simulink library "Lib_Solve_PWLinearize_TMATS"  (R2019b)
settings: Solver=ode45  StartTime=0.0  StopTime=10.0  RelTol=1e-3  EnableMultiTasking=on
libraries: simulink x8, Lib_Solve_Linearize_TMATS x1, Lib_Cntrl_SetPointCntrlPI_TMATS x1, Lib_Solve_OuterLoopIntegrator_TMATS x1
Description:
  | Thomas Modules
settings Model: Creator=jwchapm2  LastModifiedBy=bhisma
settings DataIOCC: LimitDataPoints=on  SaveFormat=Array  ReturnWorkspaceOutputs=off
settings OptimizationCC: ExpressionDepthLimit=2147483647  LifeSpan=inf
settings DebuggingCC: UnderspecifiedInitializationDetection=Classic  MergeDetectMultiDrivingBlocksExec=none  SolverPrmCheckMsg=warning  StateNameClashWarn=warning  SFUnexpectedBacktrackingDiag=warning  SFNoUnconditionalDefaultTransitionDiag=warning  SFExecutionAtInitializationDiag=none  ArithmeticOperatorsInVariantConditions=warning
settings HardwareCC: ProdBitPerPointer=32  ProdBitPerSizeT=32  ProdBitPerPtrDiffT=32  ProdLargestAtomicFloat=None  ProdIntDivRoundTo=Undefined  ProdEndianess=Unspecified  ProdWordSize=32  ProdHWDeviceType=32-bit Generic
settings ModelReferenceCC: PropagateSignalLabelsOutOfModel=off
settings SFSimCC: SimUseLocalCustomCode=off  CustomCodeUndefinedFunction=UseInterfaceOnly
settings RTWCC: RTWUseLocalCustomCode=off
settings CodeAppCC: StateflowObjectComments=on
settings GRTTargetCC: TargetLangStandard=C89/C90 (ANSI)  GeneratePreprocessorConditionals=Disable all
settings ConfigComp: CovMetricSettings=dw  CovHtmlReporting=on  CovSaveCumulativeToWorkspaceVar=on  CovSaveSingleToWorkspaceVar=on  CovExternalEMLEnable=off

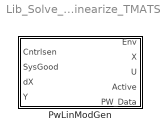
== system Lib_Solve_PWLinearize_TMATS ==
  PwLinModGen : Subsystem  mask(T-MATS: Piecewise Linear Model Generator Library Block){Env_M=[0 100 1000;0 0.05 0.1], DCntrlEn_M=off, TVec_M=0: 50: 100, XIC_M=[7000; 10000], UIC_M=10000, Ts_M=0.015, Kp_M=0.001, Ki_M=0.001, ER_M=[100; 0.001], UR_M=2, dXC_M=0.001, Fail_M=2, XPer_M=[0.01;-0.01], UPer_M=[0.01;-0.01], NY_M=8, BN_M=double(gcb)}
      mask prompts: Env_M "Env_M - Environmental Parameter Array (mxn)"; DCntrlEn_M "DCntrlEn_M - Enable direct U control"; TVec_M "TVec_M - Target control value or direct U vector (rx1)"; XIC_M "XIC_M - Initial conditions for system states (px1)"; UIC_M "UIC_M - Initial conditions for U (1x1)"; Ts_M "Ts_M - Sample time"; ER_M "ER_M - quasi-steady-state environmental parameter slew rate (mx1)"; UR_M "UR_M - quasi-steady-state U slew rate (1x1)"; dXC_M "dXC_M - dX steady-state conditional limit"; Fail_M "Fail_M - Time required to fail slew run (sec)"; XPer_M "XPer_M - X perturbation values (rxm) [frac]"; UPer_M "UPer_M - U perturbation values (rx1) [frac]"; NY_M "NY_M - Number of Y variables"; BN_M "BN_M - Block Name"
      mask help:
      | This block is meant to automatically create a piecewise linear model of a system.
      |
      | This model will be of the form:
      | (xdot - xdot_0) = A*(x - x0) + B*(u - u0)
      | (y - y0) = C*(x - x0) + D*(u - u0)
      |
      | Where x is the system state, u is the system input, and y is the plant output.
      | 0 values are the trim point values.
      |
      | This block should only be used when U is a 1x1 and the system states are external.
      |
      | During operation, the block will dynamically move or "slew" the system input and various environmental inputs to the defined operational points. At these points the block will wait for the system to reach steady state, then freeze the state integrators while the system is linearized using the perturbation method (see the T-MATS linearization block). As points are linearized, the block will output the linear models to the file "LinPW_TMATS.mat". Control of u slew rates can be managed in two ways. First with a direct dynamic slew of u (check box DCntrlEn_M) and second with by using u as an effector to meet a desired control value. The control value can be input into the Cntrlsen input and u is adjusted via a proportional integral (PI) controller to move the system to the desired control value.
      | For more information click on the help button.
      mask init:
      | if DCntrlEn_M == 0
      |     if strcmp(get_param([BN_M '/Cntrlsen'],'BlockType'),'Constant')
      |         MSK_ReplaceBlock_TMATS([BN_M '/Cntrlsen'],'built-in/Inport');
      |     end
      |     set_param([BN_M '/Cntrlsen'],'Port',num2str(1));
      | elseif DCntrlEn_M == 1
      |     if strcmp(get_param([BN_M '/Cntrlsen'],'BlockType'),'Inport')
      |         MSK_ReplaceBlock_TMATS([BN_M '/Cntrlsen'],'built-in/Constant');
      |         set_param([BN_M '/Cntrlsen'],'Value','[0]');
      |     end
      | end
      mask Help: web(which('Solver_TMATS_PWLinearize.html'),'-helpbrowser')
      mask Callback DCntrlEn_M: MSK_SEC_Enables_TMATS('DCntrlEn_M',[7,8],'dis')
      mask DialogControl Container4 Prompt: Slew
      mask DialogControl Container7 Prompt: SlewCntrl
      mask DialogControl Container5 Prompt: Linearization

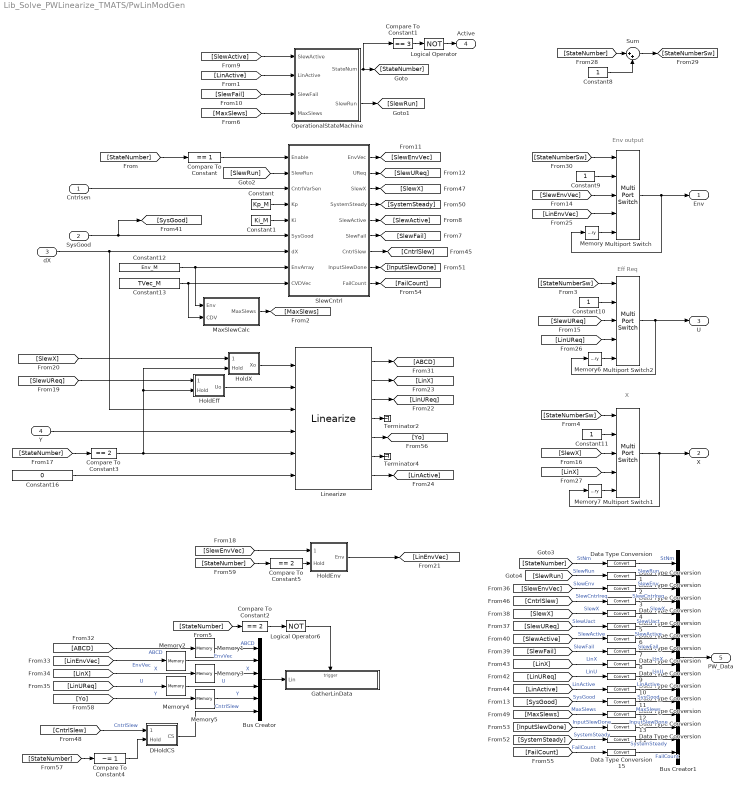
== system Lib_Solve_PWLinearize_TMATS/PwLinModGen ==
  note: X
  note: Eff Req
  note: Env output
  Cntrlsen : Inport
  SysGood : Inport  Port=2
  dX : Inport  Port=3
  Y : Inport  Port=4
  Bus Creator : BusCreator  Inputs=6
  Bus Creator1 : BusCreator  Inputs=16
  Compare To Constant : simulink/Logic and Bit Operations/Compare To Constant  relop===  const=1  OutDataTypeStr=boolean
  Compare To Constant1 : simulink/Logic and Bit Operations/Compare To Constant  relop===  const=3  OutDataTypeStr=boolean
  Compare To Constant2 : simulink/Logic and Bit Operations/Compare To Constant  relop===  const=2  OutDataTypeStr=boolean
  Compare To Constant3 : simulink/Logic and Bit Operations/Compare To Constant  relop===  const=2  OutDataTypeStr=boolean
  Compare To Constant4 : simulink/Logic and Bit Operations/Compare To Constant  relop=~=  const=1  OutDataTypeStr=boolean
  Compare To Constant5 : simulink/Logic and Bit Operations/Compare To Constant  relop===  const=2  OutDataTypeStr=boolean
  Constant : Constant  Value=Kp_M
  Constant1 : Constant  Value=Ki_M
  Constant{8..11} (4 alike) : Constant
  Constant12 : Constant  Value=Env_M
  Constant13 : Constant  Value=TVec_M
  Constant16 : Constant  Value=0
  DHoldCS : Subsystem
  Data Type Conversion{,1..15} (16 alike) : DataTypeConversion
  GatherLinData : Subsystem
  HoldEff : Subsystem
  HoldEnv : Subsystem
  HoldX : Subsystem
  Linearize : Lib_Solve_Linearize_TMATS/Linearize  N_XPer_M=XPer_M  N_UPer_M=UPer_M  N_Y_M=NY_M
  Logical Operator : Logic  Operator=NOT  AllPortsSameDT=off  OutDataTypeStr=boolean
  Logical Operator6 : Logic  Operator=NOT  AllPortsSameDT=off  OutDataTypeStr=boolean
  MaxSlewCalc : Subsystem
  Memory : Memory  InitialCondition=Env_M(:,1)
  Memory{1..5} (5 alike) : Memory
  Memory6 : Memory  InitialCondition=UIC_M
  Memory7 : Memory  InitialCondition=XIC_M
  Multiport Switch : MultiPortSwitch  Inputs=4
  Multiport Switch1 : MultiPortSwitch  Inputs=4
  Multiport Switch2 : MultiPortSwitch  Inputs=4
  OperationalStateMachine : Subsystem  TreatAsAtomicUnit=on
  SlewCntrl : Subsystem
  Sum : Sum  Inputs=|++
  Terminator2 : Terminator
  Terminator4 : Terminator
  Env : Outport  PortDimensions=size(Env_M,1)
  X : Outport  Port=2  PortDimensions=length(XIC_M)
  U : Outport  Port=3  PortDimensions=length(UIC_M)
  Active : Outport  Port=4
  PW_Data : Outport  Port=5
  wires:
  Bus Creator/1 -> GatherLinData/1(Lin)
  [LinUReq] -> Memory4/1  "U"
  [ABCD] -> Memory1/1  "ABCD"
  [LinEnvVec] -> Memory2/1  "EnvVec"
  [LinX] -> Memory3/1  "X"
  Logical Operator6/1 -> GatherLinData/Trigger
  [StateNumber] -> Compare To Constant2/1
  Compare To Constant2/1 -> Logical Operator6/1
  Logical Operator/1 -> Active/1
  Compare To Constant1/1 -> Logical Operator/1
  SlewCntrl/1(EnvVec) -> [SlewEnvVec]
  [SlewX] -> HoldX/1(SlewX)
  [StateNumber] -> Sum/1
  Memory7/1 -> Multiport Switch1/5
  Constant11/1 -> Multiport Switch1/2
  Constant10/1 -> Multiport Switch2/2
  [SlewUReq] -> Multiport Switch2/3
  Memory6/1 -> Multiport Switch2/5
  Memory/1 -> Multiport Switch/5
  [LinUReq] -> Multiport Switch2/4
  Constant9/1 -> Multiport Switch/2
  [SlewUReq] -> HoldEff/1(SlewU)
  Multiport Switch1/1 -> Memory7/1, X/1
  [StateNumber] -> Compare To Constant/1
  [StateNumberSw] -> Multiport Switch1/1
  [StateNumberSw] -> Multiport Switch2/1
  [StateNumberSw] -> Multiport Switch/1
  OperationalStateMachine/1(StateNum) -> [StateNumber], Compare To Constant1/1
  Constant13/1 -> MaxSlewCalc/2(CDV), SlewCntrl/9(CVDVec)
  Constant12/1 -> MaxSlewCalc/1(Env), SlewCntrl/8(EnvArray)
  MaxSlewCalc/1(MaxSlews) -> [MaxSlews]
  dX/1 -> Linearize/3, SlewCntrl/7(dX)
  Constant16/1 -> Linearize/6
  Y/1 -> Linearize/4
  Constant8/1 -> Sum/2
  Sum/1 -> [StateNumberSw]
  [MaxSlews] -> OperationalStateMachine/4(MaxSlews)
  Linearize/1 -> [ABCD]
  Linearize/6 -> Terminator4/1
  Linearize/5 -> [Yo]
  Linearize/4 -> Terminator2/1
  Compare To Constant3/1 -> Linearize/5, HoldX/2(Hold), HoldEff/2(Hold)
  SysGood/1 -> [SysGood], SlewCntrl/6(SysGood)
  SlewCntrl/2(UReq) -> [SlewUReq]
  [SlewActive] -> OperationalStateMachine/1(SlewActive)
  [StateNumber] -> Compare To Constant3/1
  Linearize/7 -> [LinActive]
  [LinActive] -> OperationalStateMachine/2(LinActive)
  [SlewEnvVec] -> Multiport Switch/3
  OperationalStateMachine/2(SlewRun) -> [SlewRun]
  [LinX] -> Multiport Switch1/4
  SlewCntrl/5(SlewActive) -> [SlewActive]
  Multiport Switch2/1 -> Memory6/1, U/1
  [SlewFail] -> OperationalStateMachine/3(SlewFail)
  SlewCntrl/6(SlewFail) -> [SlewFail]
  HoldEff/1(Uo) -> Linearize/2
  [SlewRun] -> SlewCntrl/2(SlewRun)
  Cntrlsen/1 -> SlewCntrl/3(CntrlVarSen)
  [SlewX] -> Multiport Switch1/3
  Constant1/1 -> SlewCntrl/5(Ki)
  SlewCntrl/4(SystemSteady) -> [SystemSteady]
  Constant/1 -> SlewCntrl/4(Kp)
  Linearize/2 -> [LinX]
  [LinEnvVec] -> Multiport Switch/4
  HoldEnv/1(Env) -> [LinEnvVec]
  Linearize/3 -> [LinUReq]
  Multiport Switch/1 -> Memory/1, Env/1
  [CntrlSlew] -> Data Type Conversion3/1  "SlewCntrlreq"
  [SlewRun] -> Data Type Conversion1/1  "SlewRun"
  [SlewEnvVec] -> Data Type Conversion2/1  "SlewEnv"
  [SlewX] -> Data Type Conversion4/1  "SlewX"
  [StateNumber] -> Data Type Conversion/1  "StNm"
  [LinX] -> Data Type Conversion8/1  "LinX"
  [SlewUReq] -> Data Type Conversion5/1  "SlewUact"
  [LinActive] -> Data Type Conversion10/1  "LinActive"
  [SlewFail] -> Data Type Conversion7/1  "SlewFail"
  [LinUReq] -> Data Type Conversion9/1  "LinU"
  [SlewActive] -> Data Type Conversion6/1  "SlewActive"
  Bus Creator1/1 -> PW_Data/1
  Compare To Constant/1 -> SlewCntrl/1(Enable)
  SlewCntrl/3(SlewX) -> [SlewX]
  [SysGood] -> Data Type Conversion11/1  "SysGood"
  [CntrlSlew] -> DHoldCS/1(CntrlSlew)  "CntrlSlew"
  [MaxSlews] -> Data Type Conversion12/1  "MaxSlews"
  SlewCntrl/8(InputSlewDone) -> [InputSlewDone]
  [InputSlewDone] -> Data Type Conversion13/1  "InputSlewDone"
  [SystemSteady] -> Data Type Conversion14/1  "SystemSteady"
  SlewCntrl/9(FailCount) -> [FailCount]
  [FailCount] -> Data Type Conversion15/1  "FailCount"
  HoldX/1(Xo) -> Linearize/1
  [Yo] -> Memory5/1  "Y"
  Memory1/1 -> Bus Creator/1  "ABCD"
  Memory2/1 -> Bus Creator/2  "EnvVec"
  Memory3/1 -> Bus Creator/3  "X"
  Memory4/1 -> Bus Creator/4  "U"
  Memory5/1 -> Bus Creator/5  "Y"
  DHoldCS/1(CS) -> Bus Creator/6  "CntrlSlew"
  SlewCntrl/7(CntrlSlew) -> [CntrlSlew]
  [StateNumber] -> Compare To Constant4/1
  Compare To Constant4/1 -> DHoldCS/2(Hold)
  Data Type Conversion/1 -> Bus Creator1/1  "StNm"
  Data Type Conversion1/1 -> Bus Creator1/2  "SlewRun"
  Data Type Conversion2/1 -> Bus Creator1/3  "SlewEnv"
  Data Type Conversion3/1 -> Bus Creator1/4  "SlewCntrlreq"
  Data Type Conversion4/1 -> Bus Creator1/5  "SlewX"
  Data Type Conversion5/1 -> Bus Creator1/6  "SlewUact"
  Data Type Conversion6/1 -> Bus Creator1/7  "SlewActive"
  Data Type Conversion7/1 -> Bus Creator1/8  "SlewFail"
  Data Type Conversion8/1 -> Bus Creator1/9  "LinX"
  Data Type Conversion9/1 -> Bus Creator1/10  "LinU"
  Data Type Conversion10/1 -> Bus Creator1/11  "LinActive"
  Data Type Conversion11/1 -> Bus Creator1/12  "SysGood"
  Data Type Conversion12/1 -> Bus Creator1/13  "MaxSlews"
  Data Type Conversion13/1 -> Bus Creator1/14  "InputSlewDone"
  Data Type Conversion14/1 -> Bus Creator1/15  "SystemSteady"
  Data Type Conversion15/1 -> Bus Creator1/16  "FailCount"
  [SlewEnvVec] -> HoldEnv/1(SlewEnv)
  [StateNumber] -> Compare To Constant5/1
  Compare To Constant5/1 -> HoldEnv/2(Hold)

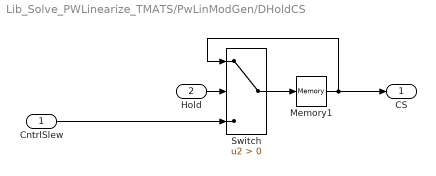
== system Lib_Solve_PWLinearize_TMATS/PwLinModGen/DHoldCS ==
  CntrlSlew : Inport
  Hold : Inport  Port=2
  Memory1 : Memory  InitialCondition=TVec_M(1)
  Switch : Switch  Criteria=u2 > Threshold
  CS : Outport
  wires:
  CntrlSlew/1 -> Switch/3
  Memory1/1 -> Switch/1, CS/1
  Hold/1 -> Switch/2
  Switch/1 -> Memory1/1

== system Lib_Solve_PWLinearize_TMATS/PwLinModGen/GatherLinData ==
  Lin : Inport
  Trigger : TriggerPort  VariantControl=(inherit)  PortDimensions=1
  To File : ToFile  Filename=LinPW_TMATS  MatrixName=LinSys  SaveFormat=Timeseries
  wires:
  Lin/1 -> To File/1

== system Lib_Solve_PWLinearize_TMATS/PwLinModGen/HoldEff ==
  SlewU : Inport
  Hold : Inport  Port=2
  Memory2 : Memory  InitialCondition=UIC_M
  Switch : Switch  Criteria=u2 > Threshold
  Uo : Outport
  wires:
  Switch/1 -> Memory2/1, Uo/1
  Hold/1 -> Switch/2
  Memory2/1 -> Switch/1
  SlewU/1 -> Switch/3

== system Lib_Solve_PWLinearize_TMATS/PwLinModGen/HoldEnv ==
  SlewEnv : Inport
  Hold : Inport  Port=2
  Memory2 : Memory  InitialCondition=Env_M(:,1)
  Switch : Switch  Criteria=u2 > Threshold
  Env : Outport
  wires:
  SlewEnv/1 -> Switch/3
  Memory2/1 -> Switch/1
  Hold/1 -> Switch/2
  Switch/1 -> Env/1, Memory2/1

== system Lib_Solve_PWLinearize_TMATS/PwLinModGen/HoldX ==
  SlewX : Inport
  Hold : Inport  Port=2
  Memory2 : Memory  InitialCondition=XIC_M
  Switch : Switch  Criteria=u2 > Threshold
  Xo : Outport
  wires:
  Memory2/1 -> Switch/1
  Hold/1 -> Switch/2
  SlewX/1 -> Switch/3
  Switch/1 -> Memory2/1, Xo/1

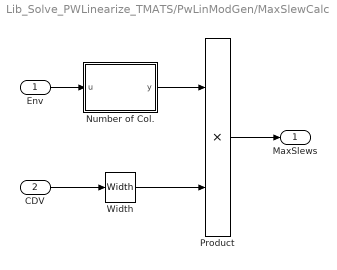
== system Lib_Solve_PWLinearize_TMATS/PwLinModGen/MaxSlewCalc ==
  Env : Inport
  CDV : Inport  Port=2
  Number of Col. : MATLAB Function  TreatAsAtomicUnit=on
  Product : Product
  Width : Width
  MaxSlews : Outport
  wires:
  CDV/1 -> Width/1
  Env/1 -> Number of Col./1(u)
  Number of Col./1(y) -> Product/1
  Product/1 -> MaxSlews/1
  Width/1 -> Product/2

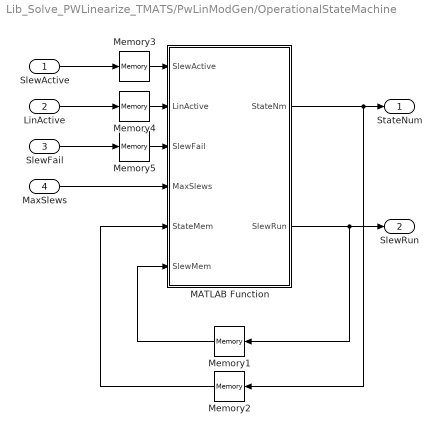
== system Lib_Solve_PWLinearize_TMATS/PwLinModGen/OperationalStateMachine ==
  SlewActive : Inport
  LinActive : Inport  Port=2
  SlewFail : Inport  Port=3
  MaxSlews : Inport  Port=4
  MATLAB Function : MATLAB Function  TreatAsAtomicUnit=on
  Memory1 : Memory  InitialCondition=1
  Memory{2..5} (4 alike) : Memory
  StateNum : Outport
  SlewRun : Outport  Port=2
  wires:
  MaxSlews/1 -> MATLAB Function/4(MaxSlews)
  Memory4/1 -> MATLAB Function/2(LinActive)
  LinActive/1 -> Memory4/1
  Memory5/1 -> MATLAB Function/3(SlewFail)
  Memory3/1 -> MATLAB Function/1(SlewActive)
  SlewFail/1 -> Memory5/1
  SlewActive/1 -> Memory3/1
  Memory1/1 -> MATLAB Function/6(SlewMem)
  MATLAB Function/2(SlewRun) -> SlewRun/1, Memory1/1
  MATLAB Function/1(StateNm) -> Memory2/1, StateNum/1
  Memory2/1 -> MATLAB Function/5(StateMem)

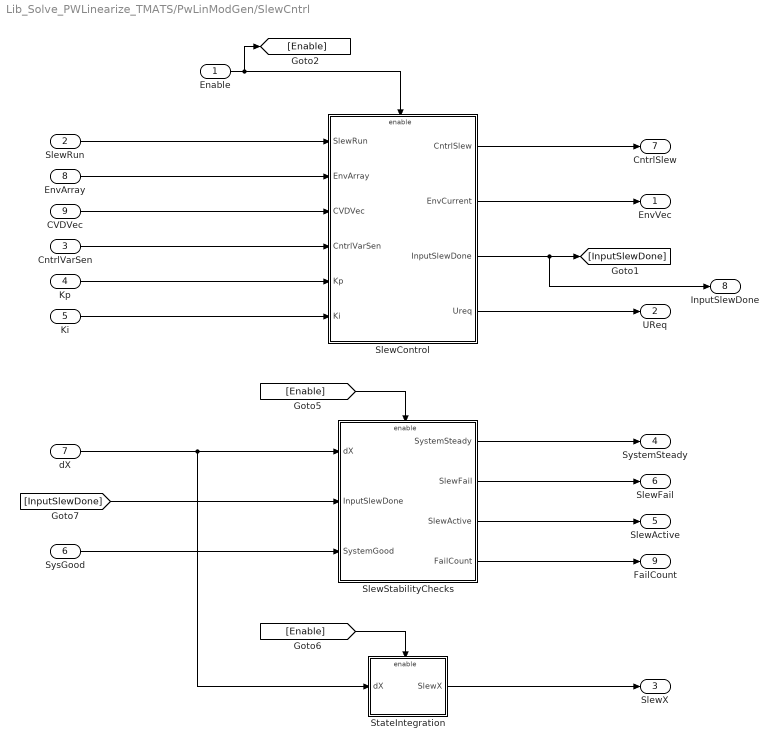
== system Lib_Solve_PWLinearize_TMATS/PwLinModGen/SlewCntrl ==
  Enable : Inport
  SlewRun : Inport  Port=2
  CntrlVarSen : Inport  Port=3
  Kp : Inport  Port=4
  Ki : Inport  Port=5
  SysGood : Inport  Port=6
  dX : Inport  Port=7
  EnvArray : Inport  Port=8
  CVDVec : Inport  Port=9
  SlewControl : Subsystem
  SlewStabilityChecks : Subsystem
  StateIntegration : Subsystem
  EnvVec : Outport
  UReq : Outport  Port=2
  SlewX : Outport  Port=3
  SystemSteady : Outport  Port=4
  SlewActive : Outport  Port=5
  SlewFail : Outport  Port=6
  CntrlSlew : Outport  Port=7
  InputSlewDone : Outport  Port=8
  FailCount : Outport  Port=9
  wires:
  SlewRun/1 -> SlewControl/1(SlewRun)
  EnvArray/1 -> SlewControl/2(EnvArray)
  CVDVec/1 -> SlewControl/3(CVDVec)
  CntrlVarSen/1 -> SlewControl/4(CntrlVarSen)
  Kp/1 -> SlewControl/5(Kp)
  Ki/1 -> SlewControl/6(Ki)
  SlewControl/1(CntrlSlew) -> CntrlSlew/1
  SlewControl/2(EnvCurrent) -> EnvVec/1
  SlewControl/3(InputSlewDone) -> InputSlewDone/1, [InputSlewDone]
  SlewControl/4(Ureq) -> UReq/1
  dX/1 -> StateIntegration/1(dX), SlewStabilityChecks/1(dX)
  [InputSlewDone] -> SlewStabilityChecks/2(InputSlewDone)
  SysGood/1 -> SlewStabilityChecks/3(SystemGood)
  SlewStabilityChecks/1(SystemSteady) -> SystemSteady/1
  SlewStabilityChecks/2(SlewFail) -> SlewFail/1
  SlewStabilityChecks/3(SlewActive) -> SlewActive/1
  Enable/1 -> SlewControl/Enable, [Enable]
  [Enable] -> SlewStabilityChecks/Enable
  [Enable] -> StateIntegration/Enable
  StateIntegration/1(SlewX) -> SlewX/1
  SlewStabilityChecks/4(FailCount) -> FailCount/1

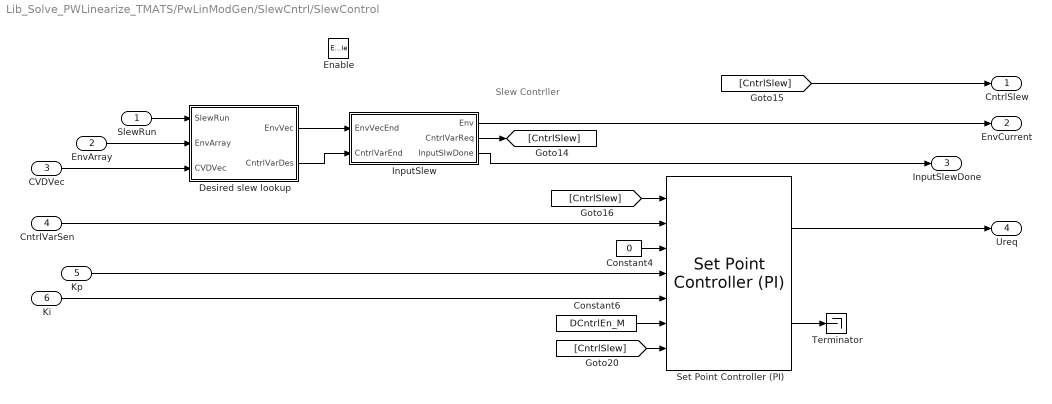
== system Lib_Solve_PWLinearize_TMATS/PwLinModGen/SlewCntrl/SlewControl ==
  note: Slew Contrller
  SlewRun : Inport
  EnvArray : Inport  Port=2
  CVDVec : Inport  Port=3
  CntrlVarSen : Inport  Port=4
  Kp : Inport  Port=5
  Ki : Inport  Port=6
  Enable : EnablePort
  Constant4 : Constant  Value=0
  Constant6 : Constant  Value=DCntrlEn_M
  Desired slew lookup : Subsystem
  InputSlew : Subsystem
  Set Point Controller (PI) : Lib_Cntrl_SetPointCntrlPI_TMATS/Set Point Controller (PI)  PI_IC_M=UIC_M  WGain_M=0  Ts_M=Ts_M
  Terminator : Terminator
  CntrlSlew : Outport
  EnvCurrent : Outport  Port=2
  InputSlewDone : Outport  Port=3
  Ureq : Outport  Port=4
  wires:
  Constant4/1 -> Set Point Controller (PI)/3
  CVDVec/1 -> Desired slew lookup/3(CVDVec)
  SlewRun/1 -> Desired slew lookup/1(SlewRun)
  Desired slew lookup/1(EnvVec) -> InputSlew/1(EnvVecEnd)
  Kp/1 -> Set Point Controller (PI)/4
  InputSlew/3(InputSlwDone) -> InputSlewDone/1
  Desired slew lookup/2(CntrlVarDes) -> InputSlew/2(CntrlVarEnd)
  CntrlVarSen/1 -> Set Point Controller (PI)/2
  Ki/1 -> Set Point Controller (PI)/5
  InputSlew/1(Env) -> EnvCurrent/1
  Set Point Controller (PI)/1 -> Ureq/1
  Constant6/1 -> Set Point Controller (PI)/6
  [CntrlSlew] -> Set Point Controller (PI)/7
  Set Point Controller (PI)/2 -> Terminator/1
  InputSlew/2(CntrlVarReq) -> [CntrlSlew]
  [CntrlSlew] -> CntrlSlew/1
  [CntrlSlew] -> Set Point Controller (PI)/1
  EnvArray/1 -> Desired slew lookup/2(EnvArray)

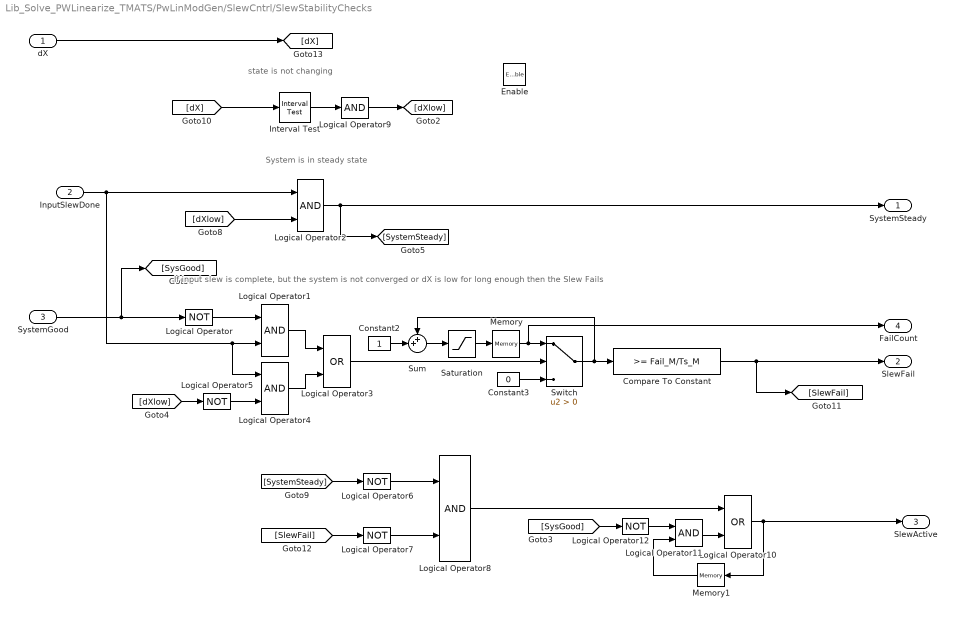
== system Lib_Solve_PWLinearize_TMATS/PwLinModGen/SlewCntrl/SlewStabilityChecks ==
  note: state is not changing
  note: If input slew is complete, but the system is not converged or dX is low for long enough then the Slew Fails
  note: System is in steady state
  dX : Inport
  InputSlewDone : Inport  Port=2
  SystemGood : Inport  Port=3
  Enable : EnablePort
  Compare To Constant : simulink/Logic and Bit Operations/Compare To Constant  relop=>=  const=Fail_M/Ts_M  OutDataTypeStr=boolean
  Constant2 : Constant
  Constant3 : Constant  Value=0
  Interval Test : simulink/Logic and Bit Operations/Interval Test  IntervalClosedRight=on  uplimit=dXC_M  IntervalClosedLeft=on  lowlimit=-dXC_M  OutDataTypeStr=boolean
  Logical Operator{,5..7,12} (5 alike) : Logic  Operator=NOT  AllPortsSameDT=off  OutDataTypeStr=boolean
  Logical Operator{1..2,4,8,11} (5 alike) : Logic  AllPortsSameDT=off  OutDataTypeStr=boolean
  Logical Operator10 : Logic  Operator=OR  AllPortsSameDT=off  OutDataTypeStr=boolean
  Logical Operator3 : Logic  Operator=OR  AllPortsSameDT=off  OutDataTypeStr=boolean
  Logical Operator9 : Logic  Inputs=1  AllPortsSameDT=off  OutDataTypeStr=boolean
  Memory : Memory
  Memory1 : Memory
  Saturation : Saturate  UpperLimit=Fail_M/Ts_M  LowerLimit=0
  Sum : Sum  Inputs=++|
  Switch : Switch  Criteria=u2 > Threshold
  SystemSteady : Outport
  SlewFail : Outport  Port=2
  SlewActive : Outport  Port=3
  FailCount : Outport  Port=4
  wires:
  Logical Operator9/1 -> [dXlow]
  dX/1 -> [dX]
  Logical Operator7/1 -> Logical Operator8/2
  [SlewFail] -> Logical Operator7/1
  [SystemSteady] -> Logical Operator6/1
  Saturation/1 -> Memory/1
  Compare To Constant/1 -> SlewFail/1, [SlewFail]
  Constant3/1 -> Switch/3
  Constant2/1 -> Sum/2
  Logical Operator3/1 -> Switch/2
  Memory/1 -> FailCount/1, Switch/1
  Sum/1 -> Saturation/1
  Switch/1 -> Sum/1, Compare To Constant/1
  Logical Operator4/1 -> Logical Operator3/2
  Logical Operator5/1 -> Logical Operator4/2
  [dXlow] -> Logical Operator5/1
  Logical Operator1/1 -> Logical Operator3/1
  Logical Operator/1 -> Logical Operator1/1
  SystemGood/1 -> [SysGood], Logical Operator/1
  InputSlewDone/1 -> Logical Operator1/2, Logical Operator4/1, Logical Operator2/1
  Interval Test/1 -> Logical Operator9/1
  Logical Operator2/1 -> SystemSteady/1, [SystemSteady]
  [dX] -> Interval Test/1
  [dXlow] -> Logical Operator2/2
  Logical Operator6/1 -> Logical Operator8/1
  Logical Operator8/1 -> Logical Operator10/1
  Memory1/1 -> Logical Operator11/2
  Logical Operator10/1 -> SlewActive/1, Memory1/1
  Logical Operator11/1 -> Logical Operator10/2
  [SysGood] -> Logical Operator12/1
  Logical Operator12/1 -> Logical Operator11/1

== system Lib_Solve_PWLinearize_TMATS/PwLinModGen/SlewCntrl/StateIntegration ==
  note: State Integration
  dX : Inport
  Enable : EnablePort
  OuterLoop integrator : Lib_Solve_OuterLoopIntegrator_TMATS/OuterLoop integrator  OL_IC_M=XIC_M
  SlewX : Outport
  wires:
  OuterLoop integrator/1 -> SlewX/1
  dX/1 -> OuterLoop integrator/1

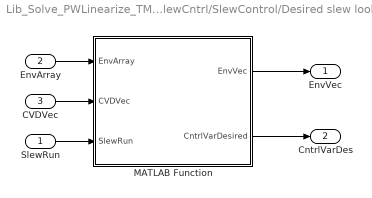
== system Lib_Solve_PWLinearize_TMATS/PwLinModGen/SlewCntrl/SlewControl/Desired slew lookup ==
  SlewRun : Inport
  EnvArray : Inport  Port=2
  CVDVec : Inport  Port=3
  MATLAB Function : MATLAB Function  TreatAsAtomicUnit=on
  EnvVec : Outport
  CntrlVarDes : Outport  Port=2
  wires:
  CVDVec/1 -> MATLAB Function/2(CVDVec)
  EnvArray/1 -> MATLAB Function/1(EnvArray)
  MATLAB Function/2(CntrlVarDesired) -> CntrlVarDes/1
  MATLAB Function/1(EnvVec) -> EnvVec/1
  SlewRun/1 -> MATLAB Function/3(SlewRun)

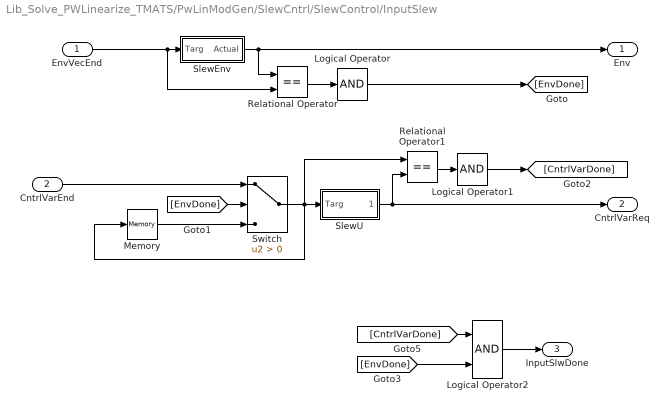
== system Lib_Solve_PWLinearize_TMATS/PwLinModGen/SlewCntrl/SlewControl/InputSlew ==
  EnvVecEnd : Inport
  CntrlVarEnd : Inport  Port=2
  Logical Operator : Logic  Inputs=1  AllPortsSameDT=off  OutDataTypeStr=boolean
  Logical Operator1 : Logic  Inputs=1  AllPortsSameDT=off  OutDataTypeStr=boolean
  Logical Operator2 : Logic  AllPortsSameDT=off  OutDataTypeStr=boolean
  Memory : Memory  InitialCondition=TVec_M(1)
  Relational Operator : RelationalOperator  Operator===  OutDataTypeStr=boolean  RndMeth=Nearest
  Relational Operator1 : RelationalOperator  Operator===  OutDataTypeStr=boolean  RndMeth=Nearest
  SlewEnv : Subsystem
  SlewU : Subsystem
  Switch : Switch  Criteria=u2 > Threshold
  Env : Outport
  CntrlVarReq : Outport  Port=2
  InputSlwDone : Outport  Port=3
  wires:
  SlewU/1(Actual) -> Relational Operator1/2, CntrlVarReq/1
  SlewEnv/1(Actual) -> Relational Operator/1, Env/1
  CntrlVarEnd/1 -> Switch/1
  Logical Operator2/1 -> InputSlwDone/1
  [EnvDone] -> Logical Operator2/2
  [CntrlVarDone] -> Logical Operator2/1
  Logical Operator1/1 -> [CntrlVarDone]
  [EnvDone] -> Switch/2
  Logical Operator/1 -> [EnvDone]
  Relational Operator1/1 -> Logical Operator1/1
  Switch/1 -> Memory/1, SlewU/1(Targ), Relational Operator1/1
  Relational Operator/1 -> Logical Operator/1
  Memory/1 -> Switch/3
  EnvVecEnd/1 -> SlewEnv/1(Targ), Relational Operator/2

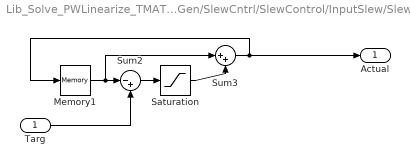
== system Lib_Solve_PWLinearize_TMATS/PwLinModGen/SlewCntrl/SlewControl/InputSlew/SlewEnv ==
  Targ : Inport
  Memory1 : Memory  InitialCondition=Env_M(:,1)
  Saturation : Saturate  UpperLimit=ER_M * Ts_M  LowerLimit=-ER_M * Ts_M
  Sum2 : Sum  Inputs=|-+
  Sum3 : Sum  Inputs=|++
  Actual : Outport
  wires:
  Saturation/1 -> Sum3/2
  Sum2/1 -> Saturation/1
  Memory1/1 -> Sum2/1, Sum3/1
  Targ/1 -> Sum2/2
  Sum3/1 -> Memory1/1, Actual/1

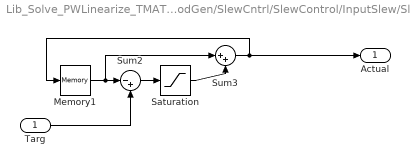
== system Lib_Solve_PWLinearize_TMATS/PwLinModGen/SlewCntrl/SlewControl/InputSlew/SlewU ==
  Targ : Inport
  Memory1 : Memory  InitialCondition=TVec_M(1)
  Saturation : Saturate  UpperLimit=UR_M * Ts_M  LowerLimit=-UR_M * Ts_M
  Sum2 : Sum  Inputs=|-+
  Sum3 : Sum  Inputs=|++
  Actual : Outport
  wires:
  Sum3/1 -> Actual/1, Memory1/1
  Targ/1 -> Sum2/2
  Memory1/1 -> Sum3/1, Sum2/1
  Sum2/1 -> Saturation/1
  Saturation/1 -> Sum3/2

== matlab function Lib_Solve_PWLinearize_TMATS/PwLinModGen/SlewCntrl/SlewControl/Desired slew lookup/MATLAB Function ==
  data: EnvArray input; CVDVec input; SlewRun input; EnvVec output; CntrlVarDesired output
function [EnvVec, CntrlVarDesired]  = fcn(EnvArray, CVDVec, SlewRun)
%#codegen

Env = EnvArray;
CVD = CVDVec;
EnvVec = Env(:,max(SlewRun-1,1)/length(CVD) +(1-rem(max(SlewRun-1,1)/length(CVD),1)));
CntrlVarDesired = CVD(rem(SlewRun-1,length(CVD))+1);

== matlab function Lib_Solve_PWLinearize_TMATS/PwLinModGen/OperationalStateMachine/MATLAB Function ==
  data: SlewActive input; LinActive input; SlewFail input; MaxSlews input; StateMem input; StateNm output; SlewRun output; SlewMem input
function [StateNm, SlewRun] = fcn(SlewActive, LinActive, SlewFail, MaxSlews, StateMem, SlewMem)
% This block defines block state transistions.

% Set State enumerations
StartSt = 0;
SlewSt = 1;
LinSt = 2;
CompletedSt = 3;

SlewRun = SlewMem;
LinDone = ~LinActive;

switch(StateMem)
    case StartSt % If this is the first run, go straight to linear model gen
        NxtSt = LinSt;
        
    case SlewSt 
        if SlewFail  % if slew failed or system is not good do not linearize and go to next slew
            SlewRun = SlewRun + 1;
            if SlewRun == MaxSlews+1
                NxtSt = CompletedSt;
            else
                NxtSt = SlewSt;
            end
            
        elseif ~SlewActive % if the slew is not active begin linearization
            NxtSt = LinSt;
            SlewRun = SlewRun + 1;
        else % if slew is active continue current slew
            NxtSt = SlewSt;
        end
        
    case LinSt % linearize and generate Kp and Ki values while active
        if LinDone && SlewRun == MaxSlews+1
            NxtSt = CompletedSt;
        elseif LinDone
            NxtSt = SlewSt;
        else
            NxtSt = LinSt;
        end
        
    case CompletedSt
        NxtSt = CompletedSt;
        
    otherwise
        NxtSt = StartSt;
        disp('Error in state processing')
end


StateNm = NxtSt;

== matlab function Lib_Solve_PWLinearize_TMATS/PwLinModGen/MaxSlewCalc/Number of Col. ==
  data: u input; y output
function y = fcn(u)
%#codegen

y = size(u,2);
